simulink model "MOBATSim"  (R2020b)
settings: Solver=FixedStepAuto  StartTime=0.0  StopTime=Sim_t  FixedStep=0.01  MinStep=0.01  RelTol=1e-2
values from neighbouring files (symbols this model uses):
  maxSpeed = car.dynamics.maxSpeed    [VehiclePathPlanner.m]    (also in VehiclePathPlanner1.m; VehiclePathPlanner_AStar.m; VehiclePathPlanner_Astar.m; VehiclePathPlanner_DStarExtraLight.m)
  Vehicles = evalin('base','Vehicles')    [Infrastructure.m]    (also in VehicleSensors.m)
undefined symbols (not defined in the file or in its folder): default_spacing, delayTimeV3, FI_distance, FI_speed, max_ac, meters, min_ac, MinDeceleration, SafeDistance, Sim_Ts, time_gap, Ts, v_set, Vehicle_id, verr_gain, vx_gain, xerr_gain
libraries: simulink x43, pid_lib x15, drivingvehiclecontroller x11, robotmobilelib x11, autolibshared x4, robotalgslib x3, mpcadaslib x1
(part 3 of 7)

== system MOBATSim/Vehicle Model 3/Safety Filter ==
  note: Longitudinal
  Reference Acceleration : Inport
  Reference Steering Angle : Inport  Port=2
  Acceleration to Speed : Integrator  LimitOutput=on  LowerSaturationLimit=0
  MATLAB System : MATLABSystem  System=VehicleSafetyFilter  Vehicle_id=Vehicle_id  SimulateUsing=Interpreted execution
      mask Type: VehicleSafetyFilter
      mask Display:
      | disp('VehicleSafetyFilter');
      | port_label('input',1,'Acc');
      | port_label('input',2,'Steering');
      | port_label('output',1,'Acc');
      | port_label('output',2,'Stop');
      | port_label('output',3,'Steering');
  Product : Product
  Signal Specification : SignalSpecification  Dimensions=1
  Stop Check : simulink/Logic and Bit Operations/Compare To Constant  relop=~=  const=1  OutDataTypeStr=uint8
  Zero-Order Hold : ZeroOrderHold  SampleTime=Sim_Ts
  Steering Angle Cmd : Outport
  Speed_input : Outport  Port=2
  wires:
  Acceleration to Speed/1 -> Signal Specification/1
  Stop Check/1 -> Product/2
  MATLAB System/3 -> Steering Angle Cmd/1
  Signal Specification/1 -> Zero-Order Hold/1
  Reference Acceleration/1 -> MATLAB System/1
  Zero-Order Hold/1 -> Product/1
  Product/1 -> Speed_input/1
  MATLAB System/1 -> Acceleration to Speed/1
  Reference Steering Angle/1 -> MATLAB System/2
  MATLAB System/2 -> Stop Check/1

== system MOBATSim/Vehicle Model 3/Transform to MOBATSim Coordinates ==
  Pose : Inport
  Constant : Constant  Value=0
  Constant1 : Constant
  Constant2 : Constant  Value=0
  Constant3 : Constant  Value=0
  Constant4 : Constant  Value=pi/2
  Gain : Gain  Gain=-1
  Matrix Concatenate : Concatenate  NumInputs=4  ConcatenateDimension=2
  Matrix Concatenate1 : Concatenate  NumInputs=3  ConcatenateDimension=2
  Selector1 : Selector  InputPortWidth=3  IndexOptions=Index vector (dialog)  Indices=[3]  OutputSizes=1
  Selector3 : Selector  InputPortWidth=3  IndexOptions=Index vector (dialog)  Indices=[1]  OutputSizes=1
  Selector4 : Selector  InputPortWidth=3  IndexOptions=Index vector (dialog)  Indices=[2]  OutputSizes=1
  Sum : Sum  Inputs=|++
  Zero-Order Hold : ZeroOrderHold  SampleTime=Sim_Ts
  Zero-Order Hold1 : ZeroOrderHold  SampleTime=Sim_Ts
  Position : Outport
  Orientation : Outport  Port=2
  wires:
  Sum/1 -> Matrix Concatenate/4
  Constant2/1 -> Matrix Concatenate/1
  Matrix Concatenate/1 -> Zero-Order Hold/1
  Constant3/1 -> Matrix Concatenate1/2
  Gain/1 -> Matrix Concatenate1/3
  Constant4/1 -> Sum/2
  Constant1/1 -> Matrix Concatenate/2
  Matrix Concatenate1/1 -> Zero-Order Hold1/1
  Selector1/1 -> Sum/1
  Constant/1 -> Matrix Concatenate/3
  Zero-Order Hold/1 -> Orientation/1
  Zero-Order Hold1/1 -> Position/1
  Selector4/1 -> Gain/1
  Selector3/1 -> Matrix Concatenate1/1
  Pose/1 -> Selector1/1, Selector4/1, Selector3/1

== system MOBATSim/Vehicle Model 3/Vehicle Model - Kinematic 3DOF Single Track ==
  WhlAngF : Inport
  xdotin : Inport  Port=2
  Bicycle Kinematic Model : robotmobilelib/Bicycle Kinematic Model  VehicleInputs=Vehicle Speed & Steering Angle  WheelBase=3  VehicleSpeedRange=[-inf inf]  MaxSteeringAngle=pi/4  InitialState=[Vehicles(Vehicle_id).dynamics.position(1); -Vehicles(Vehicle_id).dynamics.position(3);Vehicles(Vehicle_id).dynamics.orientation(4)]  SimulateUsing=Interpreted execution
      settings: SourceProductBaseCode=RO
  Delay : Delay  DelayLength=1
  Selector3 : Selector  InputPortWidth=3  IndexOptions=Index vector (dialog)  Indices=[1]  OutputSizes=1
  Selector4 : Selector  InputPortWidth=3  IndexOptions=Index vector (dialog)  Indices=[2]  OutputSizes=1
  Sqrt : Sqrt  SaturateOnIntegerOverflow=on
  Square : Math  Operator=square  SaturateOnIntegerOverflow=on
  Square1 : Math  Operator=square  SaturateOnIntegerOverflow=on
  Sum1 : Sum  Inputs=|++
  Pose : Outport
  xdot : Outport  Port=2
  wires:
  WhlAngF/1 -> Bicycle Kinematic Model/2
  xdotin/1 -> Bicycle Kinematic Model/1
  Bicycle Kinematic Model/2 -> Selector3/1, Selector4/1
  Selector3/1 -> Square/1
  Sum1/1 -> Sqrt/1
  Square1/1 -> Sum1/2
  Selector4/1 -> Square1/1
  Sqrt/1 -> Delay/1
  Square/1 -> Sum1/1
  Delay/1 -> xdot/1
  Bicycle Kinematic Model/1 -> Pose/1

== system MOBATSim/Vehicle Model 4/Longitudinal and Lateral Controllers ==
  Speed Reference : Inport
  Inter Vehicular Distance : Inport  Port=2
  Lead Speed : Inport  Port=3
  drivingMode : Inport  Port=4
  Dist2Stop : Inport  Port=5
  laneChange : Inport  Port=6
  Actual Speed : Inport  Port=7
  Actual Pose : Inport  Port=8
  Lateral Control : Subsystem
  Longitudinal Speed Control : Subsystem
  ref Acc : Outport
  ref Steering : Outport  Port=2
  wires:
  laneChange/1 -> Lateral Control/3(laneChange)
  Lateral Control/1(SteerCmd_Stanley) -> ref Steering/1
  Actual Speed/1 -> Longitudinal Speed Control/6(Actual Speed), Lateral Control/1(actualSpeed)
  drivingMode/1 -> Longitudinal Speed Control/4(Driving Mode)
  Longitudinal Speed Control/1(Longitduinal Acceleration Command) -> ref Acc/1
  Dist2Stop/1 -> Longitudinal Speed Control/5(Dist2Stop)
  Inter Vehicular Distance/1 -> Longitudinal Speed Control/2(Inter Vehicular Distance)
  Lead Speed/1 -> Longitudinal Speed Control/3(Lead Speed)
  Speed Reference/1 -> Longitudinal Speed Control/1(Speed Reference)
  Actual Pose/1 -> Lateral Control/2(actualPose)

== system MOBATSim/Vehicle Model 4/Safety Filter ==
  note: Longitudinal
  Reference Acceleration : Inport
  Reference Steering Angle : Inport  Port=2
  Acceleration to Speed : Integrator  LimitOutput=on  LowerSaturationLimit=0
  MATLAB System : MATLABSystem  System=VehicleSafetyFilter  Vehicle_id=Vehicle_id  SimulateUsing=Interpreted execution
      mask Type: VehicleSafetyFilter
      mask Display:
      | disp('VehicleSafetyFilter');
      | port_label('input',1,'Acc');
      | port_label('input',2,'Steering');
      | port_label('output',1,'Acc');
      | port_label('output',2,'Stop');
      | port_label('output',3,'Steering');
  Product : Product
  Signal Specification : SignalSpecification  Dimensions=1
  Stop Check : simulink/Logic and Bit Operations/Compare To Constant  relop=~=  const=1  OutDataTypeStr=uint8
  Zero-Order Hold : ZeroOrderHold  SampleTime=Sim_Ts
  Steering Angle Cmd : Outport
  Speed_input : Outport  Port=2
  wires:
  Acceleration to Speed/1 -> Signal Specification/1
  Stop Check/1 -> Product/2
  MATLAB System/3 -> Steering Angle Cmd/1
  Signal Specification/1 -> Zero-Order Hold/1
  Reference Acceleration/1 -> MATLAB System/1
  Zero-Order Hold/1 -> Product/1
  Product/1 -> Speed_input/1
  MATLAB System/1 -> Acceleration to Speed/1
  Reference Steering Angle/1 -> MATLAB System/2
  MATLAB System/2 -> Stop Check/1

== system MOBATSim/Vehicle Model 4/Transform to MOBATSim Coordinates ==
  Pose : Inport
  Constant : Constant  Value=0
  Constant1 : Constant
  Constant2 : Constant  Value=0
  Constant3 : Constant  Value=0
  Constant4 : Constant  Value=pi/2
  Gain : Gain  Gain=-1
  Matrix Concatenate : Concatenate  NumInputs=4  ConcatenateDimension=2
  Matrix Concatenate1 : Concatenate  NumInputs=3  ConcatenateDimension=2
  Selector1 : Selector  InputPortWidth=3  IndexOptions=Index vector (dialog)  Indices=[3]  OutputSizes=1
  Selector3 : Selector  InputPortWidth=3  IndexOptions=Index vector (dialog)  Indices=[1]  OutputSizes=1
  Selector4 : Selector  InputPortWidth=3  IndexOptions=Index vector (dialog)  Indices=[2]  OutputSizes=1
  Sum : Sum  Inputs=|++
  Zero-Order Hold : ZeroOrderHold  SampleTime=Sim_Ts
  Zero-Order Hold1 : ZeroOrderHold  SampleTime=Sim_Ts
  Position : Outport
  Orientation : Outport  Port=2
  wires:
  Sum/1 -> Matrix Concatenate/4
  Constant2/1 -> Matrix Concatenate/1
  Matrix Concatenate/1 -> Zero-Order Hold/1
  Constant3/1 -> Matrix Concatenate1/2
  Gain/1 -> Matrix Concatenate1/3
  Constant4/1 -> Sum/2
  Constant1/1 -> Matrix Concatenate/2
  Matrix Concatenate1/1 -> Zero-Order Hold1/1
  Selector1/1 -> Sum/1
  Constant/1 -> Matrix Concatenate/3
  Zero-Order Hold/1 -> Orientation/1
  Zero-Order Hold1/1 -> Position/1
  Selector4/1 -> Gain/1
  Selector3/1 -> Matrix Concatenate1/1
  Pose/1 -> Selector1/1, Selector4/1, Selector3/1

== system MOBATSim/Vehicle Model 4/Vehicle Model - Kinematic 3DOF Single Track ==
  WhlAngF : Inport
  xdotin : Inport  Port=2
  Bicycle Kinematic Model : robotmobilelib/Bicycle Kinematic Model  VehicleInputs=Vehicle Speed & Steering Angle  WheelBase=3  VehicleSpeedRange=[-inf inf]  MaxSteeringAngle=pi/4  InitialState=[Vehicles(Vehicle_id).dynamics.position(1); -Vehicles(Vehicle_id).dynamics.position(3);Vehicles(Vehicle_id).dynamics.orientation(4)]  SimulateUsing=Interpreted execution
      settings: SourceProductBaseCode=RO
  Delay : Delay  DelayLength=1
  Selector3 : Selector  InputPortWidth=3  IndexOptions=Index vector (dialog)  Indices=[1]  OutputSizes=1
  Selector4 : Selector  InputPortWidth=3  IndexOptions=Index vector (dialog)  Indices=[2]  OutputSizes=1
  Sqrt : Sqrt  SaturateOnIntegerOverflow=on
  Square : Math  Operator=square  SaturateOnIntegerOverflow=on
  Square1 : Math  Operator=square  SaturateOnIntegerOverflow=on
  Sum1 : Sum  Inputs=|++
  Pose : Outport
  xdot : Outport  Port=2
  wires:
  WhlAngF/1 -> Bicycle Kinematic Model/2
  xdotin/1 -> Bicycle Kinematic Model/1
  Bicycle Kinematic Model/2 -> Selector3/1, Selector4/1
  Selector3/1 -> Square/1
  Sum1/1 -> Sqrt/1
  Square1/1 -> Sum1/2
  Selector4/1 -> Square1/1
  Sqrt/1 -> Delay/1
  Square/1 -> Sum1/1
  Delay/1 -> xdot/1
  Bicycle Kinematic Model/1 -> Pose/1

== system MOBATSim/Vehicle Model 5/Longitudinal and Lateral Controllers ==
  Speed Reference : Inport
  Inter Vehicular Distance : Inport  Port=2
  Lead Speed : Inport  Port=3
  drivingMode : Inport  Port=4
  Dist2Stop : Inport  Port=5
  laneChange : Inport  Port=6
  Actual Speed : Inport  Port=7
  Actual Pose : Inport  Port=8
  Lateral Control : Subsystem
  Longitudinal Speed Control : Subsystem
  ref Acc : Outport
  ref Steering : Outport  Port=2
  wires:
  laneChange/1 -> Lateral Control/3(laneChange)
  Lateral Control/1(SteerCmd_Stanley) -> ref Steering/1
  Actual Speed/1 -> Longitudinal Speed Control/6(Actual Speed), Lateral Control/1(actualSpeed)
  drivingMode/1 -> Longitudinal Speed Control/4(Driving Mode)
  Longitudinal Speed Control/1(Longitduinal Acceleration Command) -> ref Acc/1
  Dist2Stop/1 -> Longitudinal Speed Control/5(Dist2Stop)
  Inter Vehicular Distance/1 -> Longitudinal Speed Control/2(Inter Vehicular Distance)
  Lead Speed/1 -> Longitudinal Speed Control/3(Lead Speed)
  Speed Reference/1 -> Longitudinal Speed Control/1(Speed Reference)
  Actual Pose/1 -> Lateral Control/2(actualPose)

== system MOBATSim/Vehicle Model 5/Safety Filter ==
  note: Longitudinal
  Reference Acceleration : Inport
  Reference Steering Angle : Inport  Port=2
  Acceleration to Speed : Integrator  LimitOutput=on  LowerSaturationLimit=0
  MATLAB System : MATLABSystem  System=VehicleSafetyFilter  Vehicle_id=Vehicle_id  SimulateUsing=Interpreted execution
      mask Type: VehicleSafetyFilter
      mask Display:
      | disp('VehicleSafetyFilter');
      | port_label('input',1,'Acc');
      | port_label('input',2,'Steering');
      | port_label('output',1,'Acc');
      | port_label('output',2,'Stop');
      | port_label('output',3,'Steering');
  Product : Product
  Signal Specification : SignalSpecification  Dimensions=1
  Stop Check : simulink/Logic and Bit Operations/Compare To Constant  relop=~=  const=1  OutDataTypeStr=uint8
  Zero-Order Hold : ZeroOrderHold  SampleTime=Sim_Ts
  Steering Angle Cmd : Outport
  Speed_input : Outport  Port=2
  wires:
  Acceleration to Speed/1 -> Signal Specification/1
  Stop Check/1 -> Product/2
  MATLAB System/3 -> Steering Angle Cmd/1
  Signal Specification/1 -> Zero-Order Hold/1
  Reference Acceleration/1 -> MATLAB System/1
  Zero-Order Hold/1 -> Product/1
  Product/1 -> Speed_input/1
  MATLAB System/1 -> Acceleration to Speed/1
  Reference Steering Angle/1 -> MATLAB System/2
  MATLAB System/2 -> Stop Check/1

== system MOBATSim/Vehicle Model 5/Transform to MOBATSim Coordinates ==
  Pose : Inport
  Constant : Constant  Value=0
  Constant1 : Constant
  Constant2 : Constant  Value=0
  Constant3 : Constant  Value=0
  Constant4 : Constant  Value=pi/2
  Gain : Gain  Gain=-1
  Matrix Concatenate : Concatenate  NumInputs=4  ConcatenateDimension=2
  Matrix Concatenate1 : Concatenate  NumInputs=3  ConcatenateDimension=2
  Selector1 : Selector  InputPortWidth=3  IndexOptions=Index vector (dialog)  Indices=[3]  OutputSizes=1
  Selector3 : Selector  InputPortWidth=3  IndexOptions=Index vector (dialog)  Indices=[1]  OutputSizes=1
  Selector4 : Selector  InputPortWidth=3  IndexOptions=Index vector (dialog)  Indices=[2]  OutputSizes=1
  Sum : Sum  Inputs=|++
  Zero-Order Hold : ZeroOrderHold  SampleTime=Sim_Ts
  Zero-Order Hold1 : ZeroOrderHold  SampleTime=Sim_Ts
  Position : Outport
  Orientation : Outport  Port=2
  wires:
  Sum/1 -> Matrix Concatenate/4
  Constant2/1 -> Matrix Concatenate/1
  Matrix Concatenate/1 -> Zero-Order Hold/1
  Constant3/1 -> Matrix Concatenate1/2
  Gain/1 -> Matrix Concatenate1/3
  Constant4/1 -> Sum/2
  Constant1/1 -> Matrix Concatenate/2
  Matrix Concatenate1/1 -> Zero-Order Hold1/1
  Selector1/1 -> Sum/1
  Constant/1 -> Matrix Concatenate/3
  Zero-Order Hold/1 -> Orientation/1
  Zero-Order Hold1/1 -> Position/1
  Selector4/1 -> Gain/1
  Selector3/1 -> Matrix Concatenate1/1
  Pose/1 -> Selector1/1, Selector4/1, Selector3/1

== system MOBATSim/Vehicle Model 5/Vehicle Model - Kinematic 3DOF Single Track ==
  WhlAngF : Inport
  xdotin : Inport  Port=2
  Bicycle Kinematic Model : robotmobilelib/Bicycle Kinematic Model  VehicleInputs=Vehicle Speed & Steering Angle  WheelBase=3  VehicleSpeedRange=[-inf inf]  MaxSteeringAngle=pi/4  InitialState=[Vehicles(Vehicle_id).dynamics.position(1); -Vehicles(Vehicle_id).dynamics.position(3);Vehicles(Vehicle_id).dynamics.orientation(4)]  SimulateUsing=Interpreted execution
      settings: SourceProductBaseCode=RO
  Delay : Delay  DelayLength=1
  Selector3 : Selector  InputPortWidth=3  IndexOptions=Index vector (dialog)  Indices=[1]  OutputSizes=1
  Selector4 : Selector  InputPortWidth=3  IndexOptions=Index vector (dialog)  Indices=[2]  OutputSizes=1
  Sqrt : Sqrt  SaturateOnIntegerOverflow=on
  Square : Math  Operator=square  SaturateOnIntegerOverflow=on
  Square1 : Math  Operator=square  SaturateOnIntegerOverflow=on
  Sum1 : Sum  Inputs=|++
  Pose : Outport
  xdot : Outport  Port=2
  wires:
  WhlAngF/1 -> Bicycle Kinematic Model/2
  xdotin/1 -> Bicycle Kinematic Model/1
  Bicycle Kinematic Model/2 -> Selector3/1, Selector4/1
  Selector3/1 -> Square/1
  Sum1/1 -> Sqrt/1
  Square1/1 -> Sum1/2
  Selector4/1 -> Square1/1
  Sqrt/1 -> Delay/1
  Square/1 -> Sum1/1
  Delay/1 -> xdot/1
  Bicycle Kinematic Model/1 -> Pose/1

== system MOBATSim/Vehicle Model 6/Longitudinal and Lateral Controllers ==
  Speed Reference : Inport
  Inter Vehicular Distance : Inport  Port=2
  Lead Speed : Inport  Port=3
  drivingMode : Inport  Port=4
  Dist2Stop : Inport  Port=5
  laneChange : Inport  Port=6
  Actual Speed : Inport  Port=7
  Actual Pose : Inport  Port=8
  Lateral Control : Subsystem
  Longitudinal Speed Control : Subsystem
  ref Acc : Outport
  ref Steering : Outport  Port=2
  wires:
  laneChange/1 -> Lateral Control/3(laneChange)
  Lateral Control/1(SteerCmd_Stanley) -> ref Steering/1
  Actual Speed/1 -> Longitudinal Speed Control/6(Actual Speed), Lateral Control/1(actualSpeed)
  drivingMode/1 -> Longitudinal Speed Control/4(Driving Mode)
  Longitudinal Speed Control/1(Longitduinal Acceleration Command) -> ref Acc/1
  Dist2Stop/1 -> Longitudinal Speed Control/5(Dist2Stop)
  Inter Vehicular Distance/1 -> Longitudinal Speed Control/2(Inter Vehicular Distance)
  Lead Speed/1 -> Longitudinal Speed Control/3(Lead Speed)
  Speed Reference/1 -> Longitudinal Speed Control/1(Speed Reference)
  Actual Pose/1 -> Lateral Control/2(actualPose)

== system MOBATSim/Vehicle Model 6/Safety Filter ==
  note: Longitudinal
  Reference Acceleration : Inport
  Reference Steering Angle : Inport  Port=2
  Acceleration to Speed : Integrator  LimitOutput=on  LowerSaturationLimit=0
  MATLAB System : MATLABSystem  System=VehicleSafetyFilter  Vehicle_id=Vehicle_id  SimulateUsing=Interpreted execution
      mask Type: VehicleSafetyFilter
      mask Display:
      | disp('VehicleSafetyFilter');
      | port_label('input',1,'Acc');
      | port_label('input',2,'Steering');
      | port_label('output',1,'Acc');
      | port_label('output',2,'Stop');
      | port_label('output',3,'Steering');
  Product : Product
  Signal Specification : SignalSpecification  Dimensions=1
  Stop Check : simulink/Logic and Bit Operations/Compare To Constant  relop=~=  const=1  OutDataTypeStr=uint8
  Zero-Order Hold : ZeroOrderHold  SampleTime=Sim_Ts
  Steering Angle Cmd : Outport
  Speed_input : Outport  Port=2
  wires:
  Acceleration to Speed/1 -> Signal Specification/1
  Stop Check/1 -> Product/2
  MATLAB System/3 -> Steering Angle Cmd/1
  Signal Specification/1 -> Zero-Order Hold/1
  Reference Acceleration/1 -> MATLAB System/1
  Zero-Order Hold/1 -> Product/1
  Product/1 -> Speed_input/1
  MATLAB System/1 -> Acceleration to Speed/1
  Reference Steering Angle/1 -> MATLAB System/2
  MATLAB System/2 -> Stop Check/1

== system MOBATSim/Vehicle Model 6/Transform to MOBATSim Coordinates ==
  Pose : Inport
  Constant : Constant  Value=0
  Constant1 : Constant
  Constant2 : Constant  Value=0
  Constant3 : Constant  Value=0
  Constant4 : Constant  Value=pi/2
  Gain : Gain  Gain=-1
  Matrix Concatenate : Concatenate  NumInputs=4  ConcatenateDimension=2
  Matrix Concatenate1 : Concatenate  NumInputs=3  ConcatenateDimension=2
  Selector1 : Selector  InputPortWidth=3  IndexOptions=Index vector (dialog)  Indices=[3]  OutputSizes=1
  Selector3 : Selector  InputPortWidth=3  IndexOptions=Index vector (dialog)  Indices=[1]  OutputSizes=1
  Selector4 : Selector  InputPortWidth=3  IndexOptions=Index vector (dialog)  Indices=[2]  OutputSizes=1
  Sum : Sum  Inputs=|++
  Zero-Order Hold : ZeroOrderHold  SampleTime=Sim_Ts
  Zero-Order Hold1 : ZeroOrderHold  SampleTime=Sim_Ts
  Position : Outport
  Orientation : Outport  Port=2
  wires:
  Sum/1 -> Matrix Concatenate/4
  Constant2/1 -> Matrix Concatenate/1
  Matrix Concatenate/1 -> Zero-Order Hold/1
  Constant3/1 -> Matrix Concatenate1/2
  Gain/1 -> Matrix Concatenate1/3
  Constant4/1 -> Sum/2
  Constant1/1 -> Matrix Concatenate/2
  Matrix Concatenate1/1 -> Zero-Order Hold1/1
  Selector1/1 -> Sum/1
  Constant/1 -> Matrix Concatenate/3
  Zero-Order Hold/1 -> Orientation/1
  Zero-Order Hold1/1 -> Position/1
  Selector4/1 -> Gain/1
  Selector3/1 -> Matrix Concatenate1/1
  Pose/1 -> Selector1/1, Selector4/1, Selector3/1

== system MOBATSim/Vehicle Model 6/Vehicle Model - Kinematic 3DOF Single Track ==
  WhlAngF : Inport
  xdotin : Inport  Port=2
  Bicycle Kinematic Model : robotmobilelib/Bicycle Kinematic Model  VehicleInputs=Vehicle Speed & Steering Angle  WheelBase=3  VehicleSpeedRange=[-inf inf]  MaxSteeringAngle=pi/4  InitialState=[Vehicles(Vehicle_id).dynamics.position(1); -Vehicles(Vehicle_id).dynamics.position(3);Vehicles(Vehicle_id).dynamics.orientation(4)]  SimulateUsing=Interpreted execution
      settings: SourceProductBaseCode=RO
  Delay : Delay  DelayLength=1
  Selector3 : Selector  InputPortWidth=3  IndexOptions=Index vector (dialog)  Indices=[1]  OutputSizes=1
  Selector4 : Selector  InputPortWidth=3  IndexOptions=Index vector (dialog)  Indices=[2]  OutputSizes=1
  Sqrt : Sqrt  SaturateOnIntegerOverflow=on
  Square : Math  Operator=square  SaturateOnIntegerOverflow=on
  Square1 : Math  Operator=square  SaturateOnIntegerOverflow=on
  Sum1 : Sum  Inputs=|++
  Pose : Outport
  xdot : Outport  Port=2
  wires:
  WhlAngF/1 -> Bicycle Kinematic Model/2
  xdotin/1 -> Bicycle Kinematic Model/1
  Bicycle Kinematic Model/2 -> Selector3/1, Selector4/1
  Selector3/1 -> Square/1
  Sum1/1 -> Sqrt/1
  Square1/1 -> Sum1/2
  Selector4/1 -> Square1/1
  Sqrt/1 -> Delay/1
  Square/1 -> Sum1/1
  Delay/1 -> xdot/1
  Bicycle Kinematic Model/1 -> Pose/1

== system MOBATSim/Vehicle Model 7/Longitudinal and Lateral Controllers ==
  Speed Reference : Inport
  Inter Vehicular Distance : Inport  Port=2
  Lead Speed : Inport  Port=3
  drivingMode : Inport  Port=4
  Dist2Stop : Inport  Port=5
  laneChange : Inport  Port=6
  Actual Speed : Inport  Port=7
  Actual Pose : Inport  Port=8
  Lateral Control : Subsystem
  Longitudinal Speed Control : Subsystem
  ref Acc : Outport
  ref Steering : Outport  Port=2
  wires:
  laneChange/1 -> Lateral Control/3(laneChange)
  Lateral Control/1(SteerCmd_Stanley) -> ref Steering/1
  Actual Speed/1 -> Longitudinal Speed Control/6(Actual Speed), Lateral Control/1(actualSpeed)
  drivingMode/1 -> Longitudinal Speed Control/4(Driving Mode)
  Longitudinal Speed Control/1(Longitduinal Acceleration Command) -> ref Acc/1
  Dist2Stop/1 -> Longitudinal Speed Control/5(Dist2Stop)
  Inter Vehicular Distance/1 -> Longitudinal Speed Control/2(Inter Vehicular Distance)
  Lead Speed/1 -> Longitudinal Speed Control/3(Lead Speed)
  Speed Reference/1 -> Longitudinal Speed Control/1(Speed Reference)
  Actual Pose/1 -> Lateral Control/2(actualPose)

== system MOBATSim/Vehicle Model 7/Safety Filter ==
  note: Longitudinal
  Reference Acceleration : Inport
  Reference Steering Angle : Inport  Port=2
  Acceleration to Speed : Integrator  LimitOutput=on  LowerSaturationLimit=0
  MATLAB System : MATLABSystem  System=VehicleSafetyFilter  Vehicle_id=Vehicle_id  SimulateUsing=Interpreted execution
      mask Type: VehicleSafetyFilter
      mask Display:
      | disp('VehicleSafetyFilter');
      | port_label('input',1,'Acc');
      | port_label('input',2,'Steering');
      | port_label('output',1,'Acc');
      | port_label('output',2,'Stop');
      | port_label('output',3,'Steering');
  Product : Product
  Signal Specification : SignalSpecification  Dimensions=1
  Stop Check : simulink/Logic and Bit Operations/Compare To Constant  relop=~=  const=1  OutDataTypeStr=uint8
  Zero-Order Hold : ZeroOrderHold  SampleTime=Sim_Ts
  Steering Angle Cmd : Outport
  Speed_input : Outport  Port=2
  wires:
  Acceleration to Speed/1 -> Signal Specification/1
  Stop Check/1 -> Product/2
  MATLAB System/3 -> Steering Angle Cmd/1
  Signal Specification/1 -> Zero-Order Hold/1
  Reference Acceleration/1 -> MATLAB System/1
  Zero-Order Hold/1 -> Product/1
  Product/1 -> Speed_input/1
  MATLAB System/1 -> Acceleration to Speed/1
  Reference Steering Angle/1 -> MATLAB System/2
  MATLAB System/2 -> Stop Check/1

== system MOBATSim/Vehicle Model 7/Transform to MOBATSim Coordinates ==
  Pose : Inport
  Constant : Constant  Value=0
  Constant1 : Constant
  Constant2 : Constant  Value=0
  Constant3 : Constant  Value=0
  Constant4 : Constant  Value=pi/2
  Gain : Gain  Gain=-1
  Matrix Concatenate : Concatenate  NumInputs=4  ConcatenateDimension=2
  Matrix Concatenate1 : Concatenate  NumInputs=3  ConcatenateDimension=2
  Selector1 : Selector  InputPortWidth=3  IndexOptions=Index vector (dialog)  Indices=[3]  OutputSizes=1
  Selector3 : Selector  InputPortWidth=3  IndexOptions=Index vector (dialog)  Indices=[1]  OutputSizes=1
  Selector4 : Selector  InputPortWidth=3  IndexOptions=Index vector (dialog)  Indices=[2]  OutputSizes=1
  Sum : Sum  Inputs=|++
  Zero-Order Hold : ZeroOrderHold  SampleTime=Sim_Ts
  Zero-Order Hold1 : ZeroOrderHold  SampleTime=Sim_Ts
  Position : Outport
  Orientation : Outport  Port=2
  wires:
  Sum/1 -> Matrix Concatenate/4
  Constant2/1 -> Matrix Concatenate/1
  Matrix Concatenate/1 -> Zero-Order Hold/1
  Constant3/1 -> Matrix Concatenate1/2
  Gain/1 -> Matrix Concatenate1/3
  Constant4/1 -> Sum/2
  Constant1/1 -> Matrix Concatenate/2
  Matrix Concatenate1/1 -> Zero-Order Hold1/1
  Selector1/1 -> Sum/1
  Constant/1 -> Matrix Concatenate/3
  Zero-Order Hold/1 -> Orientation/1
  Zero-Order Hold1/1 -> Position/1
  Selector4/1 -> Gain/1
  Selector3/1 -> Matrix Concatenate1/1
  Pose/1 -> Selector1/1, Selector4/1, Selector3/1

== system MOBATSim/Vehicle Model 7/Vehicle Model - Kinematic 3DOF Single Track ==
  WhlAngF : Inport
  xdotin : Inport  Port=2
  Bicycle Kinematic Model : robotmobilelib/Bicycle Kinematic Model  VehicleInputs=Vehicle Speed & Steering Angle  WheelBase=3  VehicleSpeedRange=[-inf inf]  MaxSteeringAngle=pi/4  InitialState=[Vehicles(Vehicle_id).dynamics.position(1); -Vehicles(Vehicle_id).dynamics.position(3);Vehicles(Vehicle_id).dynamics.orientation(4)]  SimulateUsing=Interpreted execution
      settings: SourceProductBaseCode=RO
  Delay : Delay  DelayLength=1
  Selector3 : Selector  InputPortWidth=3  IndexOptions=Index vector (dialog)  Indices=[1]  OutputSizes=1
  Selector4 : Selector  InputPortWidth=3  IndexOptions=Index vector (dialog)  Indices=[2]  OutputSizes=1
  Sqrt : Sqrt  SaturateOnIntegerOverflow=on
  Square : Math  Operator=square  SaturateOnIntegerOverflow=on
  Square1 : Math  Operator=square  SaturateOnIntegerOverflow=on
  Sum1 : Sum  Inputs=|++
  Pose : Outport
  xdot : Outport  Port=2
  wires:
  WhlAngF/1 -> Bicycle Kinematic Model/2
  xdotin/1 -> Bicycle Kinematic Model/1
  Bicycle Kinematic Model/2 -> Selector3/1, Selector4/1
  Selector3/1 -> Square/1
  Sum1/1 -> Sqrt/1
  Square1/1 -> Sum1/2
  Selector4/1 -> Square1/1
  Sqrt/1 -> Delay/1
  Square/1 -> Sum1/1
  Delay/1 -> xdot/1
  Bicycle Kinematic Model/1 -> Pose/1

== system MOBATSim/Vehicle Model 8/Longitudinal and Lateral Controllers ==
  Speed Reference : Inport
  Inter Vehicular Distance : Inport  Port=2
  Lead Speed : Inport  Port=3
  drivingMode : Inport  Port=4
  Dist2Stop : Inport  Port=5
  laneChange : Inport  Port=6
  Actual Speed : Inport  Port=7
  Actual Pose : Inport  Port=8
  Lateral Control : Subsystem
  Longitudinal Speed Control : Subsystem
  ref Acc : Outport
  ref Steering : Outport  Port=2
  wires:
  laneChange/1 -> Lateral Control/3(laneChange)
  Lateral Control/1(SteerCmd_Stanley) -> ref Steering/1
  Actual Speed/1 -> Longitudinal Speed Control/6(Actual Speed), Lateral Control/1(actualSpeed)
  drivingMode/1 -> Longitudinal Speed Control/4(Driving Mode)
  Longitudinal Speed Control/1(Longitduinal Acceleration Command) -> ref Acc/1
  Dist2Stop/1 -> Longitudinal Speed Control/5(Dist2Stop)
  Inter Vehicular Distance/1 -> Longitudinal Speed Control/2(Inter Vehicular Distance)
  Lead Speed/1 -> Longitudinal Speed Control/3(Lead Speed)
  Speed Reference/1 -> Longitudinal Speed Control/1(Speed Reference)
  Actual Pose/1 -> Lateral Control/2(actualPose)

== system MOBATSim/Vehicle Model 8/Safety Filter ==
  note: Longitudinal
  Reference Acceleration : Inport
  Reference Steering Angle : Inport  Port=2
  Acceleration to Speed : Integrator  LimitOutput=on  LowerSaturationLimit=0
  MATLAB System : MATLABSystem  System=VehicleSafetyFilter  Vehicle_id=Vehicle_id  SimulateUsing=Interpreted execution
      mask Type: VehicleSafetyFilter
      mask Display:
      | disp('VehicleSafetyFilter');
      | port_label('input',1,'Acc');
      | port_label('input',2,'Steering');
      | port_label('output',1,'Acc');
      | port_label('output',2,'Stop');
      | port_label('output',3,'Steering');
  Product : Product
  Signal Specification : SignalSpecification  Dimensions=1
  Stop Check : simulink/Logic and Bit Operations/Compare To Constant  relop=~=  const=1  OutDataTypeStr=uint8
  Zero-Order Hold : ZeroOrderHold  SampleTime=Sim_Ts
  Steering Angle Cmd : Outport
  Speed_input : Outport  Port=2
  wires:
  Acceleration to Speed/1 -> Signal Specification/1
  Stop Check/1 -> Product/2
  MATLAB System/3 -> Steering Angle Cmd/1
  Signal Specification/1 -> Zero-Order Hold/1
  Reference Acceleration/1 -> MATLAB System/1
  Zero-Order Hold/1 -> Product/1
  Product/1 -> Speed_input/1
  MATLAB System/1 -> Acceleration to Speed/1
  Reference Steering Angle/1 -> MATLAB System/2
  MATLAB System/2 -> Stop Check/1

== system MOBATSim/Vehicle Model 8/Transform to MOBATSim Coordinates ==
  Pose : Inport
  Constant : Constant  Value=0
  Constant1 : Constant
  Constant2 : Constant  Value=0
  Constant3 : Constant  Value=0
  Constant4 : Constant  Value=pi/2
  Gain : Gain  Gain=-1
  Matrix Concatenate : Concatenate  NumInputs=4  ConcatenateDimension=2
  Matrix Concatenate1 : Concatenate  NumInputs=3  ConcatenateDimension=2
  Selector1 : Selector  InputPortWidth=3  IndexOptions=Index vector (dialog)  Indices=[3]  OutputSizes=1
  Selector3 : Selector  InputPortWidth=3  IndexOptions=Index vector (dialog)  Indices=[1]  OutputSizes=1
  Selector4 : Selector  InputPortWidth=3  IndexOptions=Index vector (dialog)  Indices=[2]  OutputSizes=1
  Sum : Sum  Inputs=|++
  Zero-Order Hold : ZeroOrderHold  SampleTime=Sim_Ts
  Zero-Order Hold1 : ZeroOrderHold  SampleTime=Sim_Ts
  Position : Outport
  Orientation : Outport  Port=2
  wires:
  Sum/1 -> Matrix Concatenate/4
  Constant2/1 -> Matrix Concatenate/1
  Matrix Concatenate/1 -> Zero-Order Hold/1
  Constant3/1 -> Matrix Concatenate1/2
  Gain/1 -> Matrix Concatenate1/3
  Constant4/1 -> Sum/2
  Constant1/1 -> Matrix Concatenate/2
  Matrix Concatenate1/1 -> Zero-Order Hold1/1
  Selector1/1 -> Sum/1
  Constant/1 -> Matrix Concatenate/3
  Zero-Order Hold/1 -> Orientation/1
  Zero-Order Hold1/1 -> Position/1
  Selector4/1 -> Gain/1
  Selector3/1 -> Matrix Concatenate1/1
  Pose/1 -> Selector1/1, Selector4/1, Selector3/1

== system MOBATSim/Vehicle Model 8/Vehicle Model - Kinematic 3DOF Single Track ==
  WhlAngF : Inport
  xdotin : Inport  Port=2
  Bicycle Kinematic Model : robotmobilelib/Bicycle Kinematic Model  VehicleInputs=Vehicle Speed & Steering Angle  WheelBase=3  VehicleSpeedRange=[-inf inf]  MaxSteeringAngle=pi/4  InitialState=[Vehicles(Vehicle_id).dynamics.position(1); -Vehicles(Vehicle_id).dynamics.position(3);Vehicles(Vehicle_id).dynamics.orientation(4)]  SimulateUsing=Interpreted execution
      settings: SourceProductBaseCode=RO
  Delay : Delay  DelayLength=1
  Selector3 : Selector  InputPortWidth=3  IndexOptions=Index vector (dialog)  Indices=[1]  OutputSizes=1
  Selector4 : Selector  InputPortWidth=3  IndexOptions=Index vector (dialog)  Indices=[2]  OutputSizes=1
  Sqrt : Sqrt  SaturateOnIntegerOverflow=on
  Square : Math  Operator=square  SaturateOnIntegerOverflow=on
  Square1 : Math  Operator=square  SaturateOnIntegerOverflow=on
  Sum1 : Sum  Inputs=|++
  Pose : Outport
  xdot : Outport  Port=2
  wires:
  WhlAngF/1 -> Bicycle Kinematic Model/2
  xdotin/1 -> Bicycle Kinematic Model/1
  Bicycle Kinematic Model/2 -> Selector3/1, Selector4/1
  Selector3/1 -> Square/1
  Sum1/1 -> Sqrt/1
  Square1/1 -> Sum1/2
  Selector4/1 -> Square1/1
  Sqrt/1 -> Delay/1
  Square/1 -> Sum1/1
  Delay/1 -> xdot/1
  Bicycle Kinematic Model/1 -> Pose/1

== system MOBATSim/Vehicle Model 9/Longitudinal and Lateral Controllers ==
  Speed Reference : Inport
  Inter Vehicular Distance : Inport  Port=2
  Lead Speed : Inport  Port=3
  drivingMode : Inport  Port=4
  Dist2Stop : Inport  Port=5
  laneChange : Inport  Port=6
  Actual Speed : Inport  Port=7
  Actual Pose : Inport  Port=8
  Lateral Control : Subsystem
  Longitudinal Speed Control : Subsystem
  ref Acc : Outport
  ref Steering : Outport  Port=2
  wires:
  laneChange/1 -> Lateral Control/3(laneChange)
  Lateral Control/1(SteerCmd_Stanley) -> ref Steering/1
  Actual Speed/1 -> Longitudinal Speed Control/6(Actual Speed), Lateral Control/1(actualSpeed)
  drivingMode/1 -> Longitudinal Speed Control/4(Driving Mode)
  Longitudinal Speed Control/1(Longitduinal Acceleration Command) -> ref Acc/1
  Dist2Stop/1 -> Longitudinal Speed Control/5(Dist2Stop)
  Inter Vehicular Distance/1 -> Longitudinal Speed Control/2(Inter Vehicular Distance)
  Lead Speed/1 -> Longitudinal Speed Control/3(Lead Speed)
  Speed Reference/1 -> Longitudinal Speed Control/1(Speed Reference)
  Actual Pose/1 -> Lateral Control/2(actualPose)

== system MOBATSim/Vehicle Model 9/Safety Filter ==
  note: Longitudinal
  Reference Acceleration : Inport
  Reference Steering Angle : Inport  Port=2
  Acceleration to Speed : Integrator  LimitOutput=on  LowerSaturationLimit=0
  MATLAB System : MATLABSystem  System=VehicleSafetyFilter  Vehicle_id=Vehicle_id  SimulateUsing=Interpreted execution
      mask Type: VehicleSafetyFilter
      mask Display:
      | disp('VehicleSafetyFilter');
      | port_label('input',1,'Acc');
      | port_label('input',2,'Steering');
      | port_label('output',1,'Acc');
      | port_label('output',2,'Stop');
      | port_label('output',3,'Steering');
  Product : Product
  Signal Specification : SignalSpecification  Dimensions=1
  Stop Check : simulink/Logic and Bit Operations/Compare To Constant  relop=~=  const=1  OutDataTypeStr=uint8
  Zero-Order Hold : ZeroOrderHold  SampleTime=Sim_Ts
  Steering Angle Cmd : Outport
  Speed_input : Outport  Port=2
  wires:
  Acceleration to Speed/1 -> Signal Specification/1
  Stop Check/1 -> Product/2
  MATLAB System/3 -> Steering Angle Cmd/1
  Signal Specification/1 -> Zero-Order Hold/1
  Reference Acceleration/1 -> MATLAB System/1
  Zero-Order Hold/1 -> Product/1
  Product/1 -> Speed_input/1
  MATLAB System/1 -> Acceleration to Speed/1
  Reference Steering Angle/1 -> MATLAB System/2
  MATLAB System/2 -> Stop Check/1

== system MOBATSim/Vehicle Model 9/Transform to MOBATSim Coordinates ==
  Pose : Inport
  Constant : Constant  Value=0
  Constant1 : Constant
  Constant2 : Constant  Value=0
  Constant3 : Constant  Value=0
  Constant4 : Constant  Value=pi/2
  Gain : Gain  Gain=-1
  Matrix Concatenate : Concatenate  NumInputs=4  ConcatenateDimension=2
  Matrix Concatenate1 : Concatenate  NumInputs=3  ConcatenateDimension=2
  Selector1 : Selector  InputPortWidth=3  IndexOptions=Index vector (dialog)  Indices=[3]  OutputSizes=1
  Selector3 : Selector  InputPortWidth=3  IndexOptions=Index vector (dialog)  Indices=[1]  OutputSizes=1
  Selector4 : Selector  InputPortWidth=3  IndexOptions=Index vector (dialog)  Indices=[2]  OutputSizes=1
  Sum : Sum  Inputs=|++
  Zero-Order Hold : ZeroOrderHold  SampleTime=Sim_Ts
  Zero-Order Hold1 : ZeroOrderHold  SampleTime=Sim_Ts
  Position : Outport
  Orientation : Outport  Port=2
  wires:
  Sum/1 -> Matrix Concatenate/4
  Constant2/1 -> Matrix Concatenate/1
  Matrix Concatenate/1 -> Zero-Order Hold/1
  Constant3/1 -> Matrix Concatenate1/2
  Gain/1 -> Matrix Concatenate1/3
  Constant4/1 -> Sum/2
  Constant1/1 -> Matrix Concatenate/2
  Matrix Concatenate1/1 -> Zero-Order Hold1/1
  Selector1/1 -> Sum/1
  Constant/1 -> Matrix Concatenate/3
  Zero-Order Hold/1 -> Orientation/1
  Zero-Order Hold1/1 -> Position/1
  Selector4/1 -> Gain/1
  Selector3/1 -> Matrix Concatenate1/1
  Pose/1 -> Selector1/1, Selector4/1, Selector3/1

== system MOBATSim/Vehicle Model 9/Vehicle Model - Kinematic 3DOF Single Track ==
  WhlAngF : Inport
  xdotin : Inport  Port=2
  Bicycle Kinematic Model : robotmobilelib/Bicycle Kinematic Model  VehicleInputs=Vehicle Speed & Steering Angle  WheelBase=3  VehicleSpeedRange=[-inf inf]  MaxSteeringAngle=pi/4  InitialState=[Vehicles(Vehicle_id).dynamics.position(1); -Vehicles(Vehicle_id).dynamics.position(3);Vehicles(Vehicle_id).dynamics.orientation(4)]  SimulateUsing=Interpreted execution
      settings: SourceProductBaseCode=RO
  Delay : Delay  DelayLength=1
  Selector3 : Selector  InputPortWidth=3  IndexOptions=Index vector (dialog)  Indices=[1]  OutputSizes=1
  Selector4 : Selector  InputPortWidth=3  IndexOptions=Index vector (dialog)  Indices=[2]  OutputSizes=1
  Sqrt : Sqrt  SaturateOnIntegerOverflow=on
  Square : Math  Operator=square  SaturateOnIntegerOverflow=on
  Square1 : Math  Operator=square  SaturateOnIntegerOverflow=on
  Sum1 : Sum  Inputs=|++
  Pose : Outport
  xdot : Outport  Port=2
  wires:
  WhlAngF/1 -> Bicycle Kinematic Model/2
  xdotin/1 -> Bicycle Kinematic Model/1
  Bicycle Kinematic Model/2 -> Selector3/1, Selector4/1
  Selector3/1 -> Square/1
  Sum1/1 -> Sqrt/1
  Square1/1 -> Sum1/2
  Selector4/1 -> Square1/1
  Sqrt/1 -> Delay/1
  Square/1 -> Sum1/1
  Delay/1 -> xdot/1
  Bicycle Kinematic Model/1 -> Pose/1

== system MOBATSim/MOBATSim Library/Old Vehicle 3 Dynamic Bicycle Model with Pure Pursuit/Longitudinal Speed Control ==
  note: The vehicle calculates the speed difference between the actual speed and the reference speed, then generates the acceleration command accordingly.
  Speed Reference : Inport
  Inter Vehicular Distance : Inport  Port=2
  Lead Speed : Inport  Port=3
  Driving Mode : Inport  Port=4
  Dist2Stop : Inport  Port=5
  Actual Speed : Inport  Port=6
  Distance to Stop Controller : Subsystem
  Platoon Controller : Subsystem
  Reference Acceleration Generation : Subsystem
  Reference speed according to the driving mode : Subsystem
  Signal Specification1 : SignalSpecification  Dimensions=1
  Sum13 : Sum  Inputs=|+-
  Time Delay fault injection : Subsystem
  Vehicle Acceleration Model : Subsystem
  Longitduinal Acceleration Command : Outport  VectorParamsAs1DForOutWhenUnconnected=off
  wires:
  Platoon Controller/1(ref speed) -> Distance to Stop Controller/1(Speed Ref from Platoon), Reference speed according to the driving mode/3(2)
  Lead Speed/1 -> Platoon Controller/2(Lead Speed)
  Signal Specification1/1 -> Longitduinal Acceleration Command/1
  Sum13/1 -> Reference Acceleration Generation/2(Speed Error)
  Inter Vehicular Distance/1 -> Platoon Controller/1(Inter Vehicular Distance)
  Dist2Stop/1 -> Distance to Stop Controller/2(Distance to Stop)
  Speed Reference/1 -> Reference speed according to the driving mode/2(1)
  Distance to Stop Controller/1(ref speed) -> Reference speed according to the driving mode/4(4)
  Reference speed according to the driving mode/1(Reference Speed) -> Sum13/1
  Vehicle Acceleration Model/1(Acceleration Command) -> Signal Specification1/1
  Reference Acceleration Generation/1(Reference Acceleration Command) -> Vehicle Acceleration Model/1(Reference Acceleration Command)
  Actual Speed/1 -> Reference Acceleration Generation/3(Actual Speed), Sum13/2, Platoon Controller/3(Vehicle Speed)
  Time Delay fault injection/1(Out1) -> Reference Acceleration Generation/1(Driving Mode), Reference speed according to the driving mode/1(Driving Mode)
  Driving Mode/1 -> Time Delay fault injection/1(In1)

== system MOBATSim/MOBATSim Library/Old Vehicle 3 Dynamic Bicycle Model with Pure Pursuit/Reference Waypoint Generation ==
  Xpos : Inport
  Ypos : Inport  Port=2
  Psi : Inport  Port=3
  Speed : Inport  Port=4
  drivingMode : Inport  Port=5
  Bus Creator : BusCreator  Inputs=3
  Constant : Constant  Value=0
  Pure Pursuit : robotalgslib/Pure Pursuit  DesiredLinearVelocity=0.1  MaxAngularVelocity=1.0  LookaheadDistance=20  TargetDirPort=on  SimulateUsing=Code generation
  Terminator{,1..3} (4 alike) : Terminator
  Waypoint Generator : MATLABSystem  System=V_WPGenerator_PurePursuit  Vehicle_id=Vehicle_id  SimulateUsing=Interpreted execution
      mask Type: V_WPGenerator_PurePursuit
      mask Display:
      | disp('V_WPGenerator_PurePursuit');
      | port_label('input',1,'pose');
      | port_label('input',2,'speed');
      | port_label('output',1,'position');
      | port_label('output',2,'referenceWaypoints');
  Target Direction : Outport
  wires:
  Xpos/1 -> Bus Creator/1
  Ypos/1 -> Bus Creator/2
  Bus Creator/1 -> Waypoint Generator/1
  Psi/1 -> Bus Creator/3
  Waypoint Generator/1 -> Pure Pursuit/1
  Waypoint Generator/2 -> Pure Pursuit/2
  Pure Pursuit/1 -> Terminator/1
  Pure Pursuit/2 -> Terminator1/1
  Pure Pursuit/3 -> Target Direction/1
  Speed/1 -> Waypoint Generator/2
  drivingMode/1 -> Terminator2/1
  Constant/1 -> Terminator3/1

== system MOBATSim/MOBATSim Library/Old Vehicle 3 Dynamic Bicycle Model with Pure Pursuit/Vehicle Dynamics Interface ==
  note: Longitudinal
  note: Lateral
  Acceleration : Inport
  CollisionStatus : Inport  Port=2
  Target Direction : Inport  Port=3
  Acceleration to Speed : Integrator  LimitOutput=on  LowerSaturationLimit=0
  Collision Check : simulink/Logic and Bit Operations/Compare To Constant  relop=~=  const=3  OutDataTypeStr=uint8
  Product : Product
  Product1 : Product
  Signal Specification : SignalSpecification  Dimensions=1
  Wheel Steering Angle Formulation : Subsystem
  Zero-Order Hold : ZeroOrderHold  SampleTime=Sim_Ts
  Actual Steering Angle : Outport
  Actual Speed : Outport  Port=2
  wires:
  Zero-Order Hold/1 -> Product/1
  CollisionStatus/1 -> Collision Check/1
  Acceleration to Speed/1 -> Signal Specification/1
  Acceleration/1 -> Acceleration to Speed/1
  Signal Specification/1 -> Zero-Order Hold/1
  Collision Check/1 -> Product1/1, Product/2
  Product/1 -> Actual Speed/1
  Target Direction/1 -> Wheel Steering Angle Formulation/1(alpha)
  Product1/1 -> Actual Steering Angle/1
  Wheel Steering Angle Formulation/1(referenceYawAngle) -> Product1/2

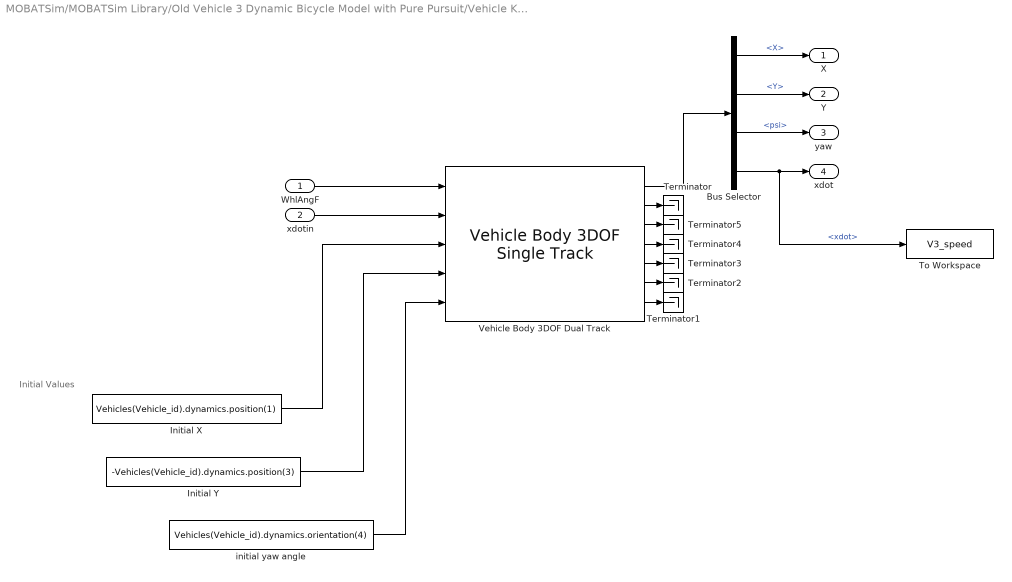
== system MOBATSim/MOBATSim Library/Old Vehicle 3 Dynamic Bicycle Model with Pure Pursuit/Vehicle Kinematic 3DOF Single Track ==
  note: Initial Values
  WhlAngF : Inport
  xdotin : Inport  Port=2
  Bus Selector : BusSelector  OutputSignals=InertFrm.Cg.Disp.X,InertFrm.Cg.Disp.Y,InertFrm.Cg.Ang.psi,BdyFrm.Cg.Vel.xdot
  Initial X : Constant  Value=Vehicles(Vehicle_id).dynamics.position(1)
  Initial Y : Constant  Value=-Vehicles(Vehicle_id).dynamics.position(3)
  Terminator{,1..5} (6 alike) : Terminator
  To Workspace : ToWorkspace  VariableName=V3_speed  SaveFormat=Timeseries  SampleTime=Sim_Ts
  Vehicle Body 3DOF Dual Track : autolibshared/Vehicle Body 3DOF Single Track  trackMode=Single (bicycle)  inputMode=External longitudinal velocity  frontSteerMode=on  rearSteerMode=off  windMode=off  muMode=off  extFMode=off  extMMode=off  htchFMode=off  htchMMode=off  extXo=on  extpsio=on  extxdoto=off  extro=off  extYo=on  extTamb=off  extydoto=off  aMode=2  NF=2  NR=2  m=2000  a=1.4  b=1.6  h=0.35  dh=1  hh=0.2  X_o=0  xdot_o=0  CalphaMode=off  sigmaMode=on  d=0  hl=0  w=[1.4,1.4]  Cy_f=12e3  Cy_r=11e3  sigma_f=.1  sigma_r=.1  alpha_f_brk=[-.1 .1]  Cy_f_data=[-9e3 9e3]  alpha_r_brk=[-.1 .1]  Cy_r_data=[-9e3 9e3]  Y_o=0  ydot_o=0  Izz=4000  psi_o=0  r_o=0  Af=2  Cd=.3  Cl=.1  Cpm=.1  beta_w=[0:0.01:0.3]  Cs=[0:0.03:0.9]  Cym=[0:0.01:0.3]  Pabs=101325  Tair=273  g=9.81  mu=1  xdot_tol=.01  Fznom=5000  Fxtire_sat=7e4  Fytire_sat=7e4  longOff=0  latOff=0  vertOff=0  wrapAng=off
      settings: SourceProductBaseCode=PW,MT,UV,VE,VP
  initial yaw angle : Constant  Value=Vehicles(Vehicle_id).dynamics.orientation(4)
  X : Outport
  Y : Outport  Port=2
  yaw : Outport  Port=3
  xdot : Outport  Port=4
  wires:
  Bus Selector/2 -> Y/1  "<Y>"
  Bus Selector/3 -> yaw/1  "<psi>"
  Bus Selector/1 -> X/1  "<X>"
  xdotin/1 -> Vehicle Body 3DOF Dual Track/2
  WhlAngF/1 -> Vehicle Body 3DOF Dual Track/1
  Initial Y/1 -> Vehicle Body 3DOF Dual Track/4
  Initial X/1 -> Vehicle Body 3DOF Dual Track/3
  initial yaw angle/1 -> Vehicle Body 3DOF Dual Track/5
  Vehicle Body 3DOF Dual Track/1 -> Bus Selector/1
  Bus Selector/4 -> To Workspace/1, xdot/1  "<xdot>"
  Vehicle Body 3DOF Dual Track/2 -> Terminator/1
  Vehicle Body 3DOF Dual Track/7 -> Terminator1/1
  Vehicle Body 3DOF Dual Track/6 -> Terminator2/1
  Vehicle Body 3DOF Dual Track/5 -> Terminator3/1
  Vehicle Body 3DOF Dual Track/4 -> Terminator4/1
  Vehicle Body 3DOF Dual Track/3 -> Terminator5/1

== system MOBATSim/MOBATSim Library/Old Vehicle 5 Dual Track/Longitudinal Speed Control ==
  note: The vehicle calculates the speed difference between the actual speed and the reference speed, then generates the acceleration command accordingly.
  Speed Reference : Inport
  Inter Vehicular Distance : Inport  Port=2
  Lead Speed : Inport  Port=3
  Driving Mode : Inport  Port=4
  Dist2Stop : Inport  Port=5
  Actual Speed : Inport  Port=6
  Distance to Stop Controller : Subsystem
  Platoon Controller : Subsystem
  Reference Acceleration Generation : Subsystem
  Reference speed according to the driving mode : Subsystem
  Signal Specification1 : SignalSpecification  Dimensions=1
  Sum13 : Sum  Inputs=|+-
  Vehicle Acceleration Model : Subsystem
  Longitduinal Acceleration Command : Outport  VectorParamsAs1DForOutWhenUnconnected=off
  wires:
  Platoon Controller/1(ref speed) -> Distance to Stop Controller/1(Speed Ref from Platoon), Reference speed according to the driving mode/3(2)
  Lead Speed/1 -> Platoon Controller/2(Lead Speed)
  Driving Mode/1 -> Reference Acceleration Generation/1(Driving Mode), Reference speed according to the driving mode/1(Driving Mode)
  Signal Specification1/1 -> Longitduinal Acceleration Command/1
  Sum13/1 -> Reference Acceleration Generation/2(Speed Error)
  Inter Vehicular Distance/1 -> Platoon Controller/1(Inter Vehicular Distance)
  Dist2Stop/1 -> Distance to Stop Controller/2(Distance to Stop)
  Speed Reference/1 -> Reference speed according to the driving mode/2(1)
  Distance to Stop Controller/1(ref speed) -> Reference speed according to the driving mode/4(4)
  Reference speed according to the driving mode/1(Reference Speed) -> Sum13/1
  Vehicle Acceleration Model/1(Acceleration Command) -> Signal Specification1/1
  Reference Acceleration Generation/1(Reference Acceleration Command) -> Vehicle Acceleration Model/1(Reference Acceleration Command)
  Actual Speed/1 -> Reference Acceleration Generation/3(Actual Speed), Sum13/2, Platoon Controller/3(Vehicle Speed)

== system MOBATSim/MOBATSim Library/Old Vehicle 5 Dual Track/Reference Waypoint Generation ==
  Xpos : Inport
  Ypos : Inport  Port=2
  Psi : Inport  Port=3
  Speed : Inport  Port=4
  drivingMode : Inport  Port=5
  Bus Creator : BusCreator  Inputs=3
  Constant : Constant  Value=0
  Constant5 : Constant
  Lateral Controller Stanley : drivingvehiclecontroller/Lateral Controller Stanley  ModelType=Kinematic bicycle model  PositionGainF=2.5  PositionGainR=2.5  YawRateGain=0.2  DelayGain=0.2  VehicleMass=1575  Lf=1.2  Lr=1.6  TireStiffness=19000  Wheelbase=3  MaxSteeringAngle=35
      settings: SourceProductBaseCode=DR
  MATLAB System : MATLABSystem  System=V_WPGenerator_Stanley  Vehicle_id=Vehicle_id  SimulateUsing=Interpreted execution
      mask Type: V_WPGenerator_Stanley
      mask Display:
      | image('WaypointGenerator.png');
      | port_label('input',1,'pose');
      | port_label('input',2,'speed');
      | port_label('input',3,'changeLane');
      | port_label('output',1,'poseOut');
      | port_label('output',2,'referencePose');
  Terminator : Terminator
  SteerCmd_Stanley : Outport
  wires:
  Xpos/1 -> Bus Creator/1
  Ypos/1 -> Bus Creator/2
  Bus Creator/1 -> MATLAB System/1
  Psi/1 -> Bus Creator/3
  MATLAB System/1 -> Lateral Controller Stanley/2
  Speed/1 -> Lateral Controller Stanley/3, MATLAB System/2
  Constant5/1 -> Lateral Controller Stanley/4
  MATLAB System/2 -> Lateral Controller Stanley/1
  Lateral Controller Stanley/1 -> SteerCmd_Stanley/1
  drivingMode/1 -> Terminator/1
  Constant/1 -> MATLAB System/3

== system MOBATSim/MOBATSim Library/Old Vehicle 5 Dual Track/Vehicle Dynamics Interface ==
  note: Longitudinal
  note: Lateral
  Acceleration : Inport
  CollisionStatus : Inport  Port=2
  SteerCmd_Stanley : Inport  Port=3
  Acceleration to Speed : Integrator  LimitOutput=on  LowerSaturationLimit=0
  Collision Check : simulink/Logic and Bit Operations/Compare To Constant  relop=~=  const=3  OutDataTypeStr=uint8
  Gain2 : Gain  Gain=pi/180
  Matrix Concatenate : Concatenate  Mode=Multidimensional array  ConcatenateDimension=2
  Product : Product
  Product1 : Product
  Signal Specification : SignalSpecification  Dimensions=1
  Zero-Order Hold : ZeroOrderHold  SampleTime=Sim_Ts
  Actual Steering Angle : Outport
  Actual Speed : Outport  Port=2
  wires:
  Zero-Order Hold/1 -> Product/1
  CollisionStatus/1 -> Collision Check/1
  Acceleration to Speed/1 -> Signal Specification/1
  Acceleration/1 -> Acceleration to Speed/1
  Signal Specification/1 -> Zero-Order Hold/1
  Collision Check/1 -> Product1/1, Product/2
  Product/1 -> Actual Speed/1
  Product1/1 -> Actual Steering Angle/1
  SteerCmd_Stanley/1 -> Gain2/1
  Gain2/1 -> Matrix Concatenate/1, Matrix Concatenate/2
  Matrix Concatenate/1 -> Product1/2
